simulink model "TemperatureControlledSystem"  (R2023b)
settings: Solver=FixedStepAuto  StartTime=0.0  StopTime=100  FixedStep=0.001  RelTol=1e-3
values from neighbouring files (symbols this model uses):
  TEMPMAX = 25.0    [temperatureControlledSystem.sldd]
  TEMPMIN = 10.0    [temperatureControlledSystem.sldd]
  TIMER = 5.0    [temperatureControlledSystem.sldd]
settings Model: DataDictionary=temperatureControlledSystem.sldd  Creator=dhabe  LastModifiedBy=dhabe
settings OptimizationCC: DefaultParameterBehavior=Inlined  EnhancedBackFolding=on  PassReuseOutputArgsAs=Individual arguments  ZeroExternalMemoryAtStartup=off  ZeroInternalMemoryAtStartup=off  OptimizeBlockOrder=speed  DifferentSizesBufferReuse=on  OptimizationCustomize=off  EfficientTunableParamExpr=on
settings DebuggingCC: ParameterTunabilityLossMsg=error
settings HardwareCC: ProdBitPerPointer=32  ProdBitPerSizeT=32  ProdBitPerPtrDiffT=32  ProdLargestAtomicFloat=None  ProdWordSize=32  ProdHWDeviceType=Atmel->AVR (32-bit)
settings SFSimCC: MATLABDynamicMemAlloc=off
settings RTWCC: Description=Embedded Coder  SystemTargetFile=ert.tlc  PackageGeneratedCodeAndArtifacts=on  TemplateMakefile=ert_default_tmf  PortableWordSizes=on
settings CodeAppCC: ForceParamTrailComments=on  IgnoreCustomStorageClasses=off  OperatorAnnotations=on  SimulinkDataObjDesc=on  SFDataObjDesc=on  InsertBlockDesc=on
settings ERTTargetCC: TargetLangStandard=C99 (ISO)  GenerateSampleERTMain=on  InlinedParameterPlacement=NonHierarchical  ERTCustomFileTemplate=example_file_process.tlc
settings ConfigComp: CovMetricSettings=dcmwe

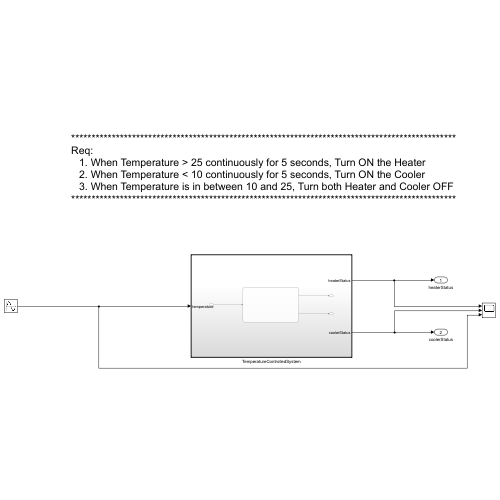
[thumbnail: Simulink's stored preview of the top-level diagram]
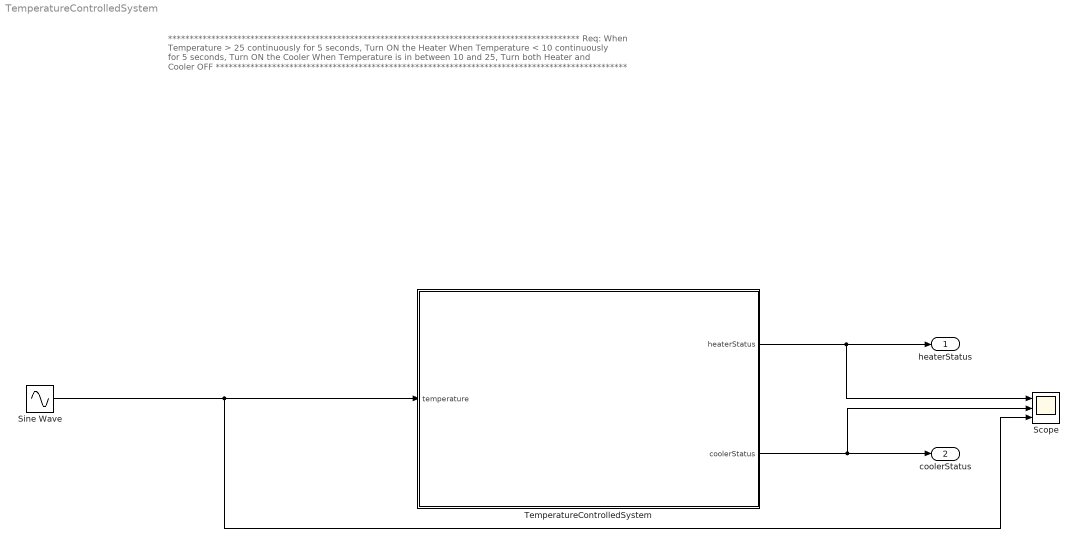
== system TemperatureControlledSystem ==
  note: ***********************************************************************************************
      | Req:
      | When Temperature > 25 continuously for 5 seconds, Turn ON the Heater
      | When Temperature < 10 continuously for 5 seconds, Turn ON the Cooler
      | When Temperature is in between 10 and 25, Turn both Heater and Cooler OFF
      | ***********************************************************************************************
  Scope : Scope  NumInputPorts=3
  Sine Wave : Sin  Amplitude=30  Frequency=0.1  SampleTime=0
  TemperatureControlledSystem : Subsystem  TreatAsAtomicUnit=on
  heaterStatus : Outport
  coolerStatus : Outport  Port=2
  wires:
  TemperatureControlledSystem/1(heaterStatus) -> Scope/1, heaterStatus/1
  TemperatureControlledSystem/2(coolerStatus) -> Scope/2, coolerStatus/1
  Sine Wave/1 -> Scope/3, TemperatureControlledSystem/1(temperature)

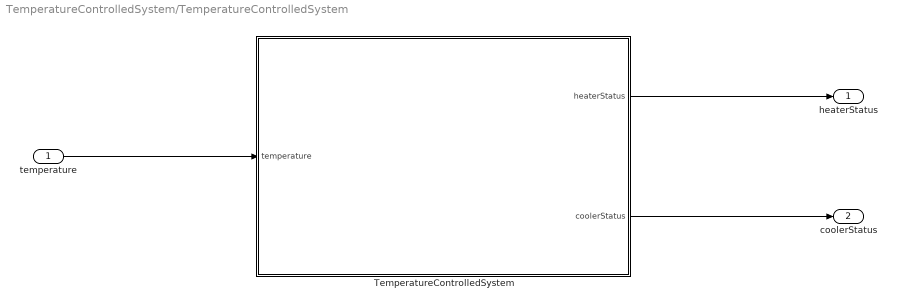
== system TemperatureControlledSystem/TemperatureControlledSystem ==
  temperature : Inport
  TemperatureControlledSystem : Stateflow chart  TreatAsAtomicUnit=on
  heaterStatus : Outport
  coolerStatus : Outport  Port=2
  wires:
  TemperatureControlledSystem/2(coolerStatus) -> coolerStatus/1
  temperature/1 -> TemperatureControlledSystem/1(temperature)
  TemperatureControlledSystem/1(heaterStatus) -> heaterStatus/1

== stateflow chart TemperatureControlledSystem/TemperatureControlledSystem ==
  settings: executeAtInitialization=1
  note: OFF = 0, ON = 1, TEMPMIN = 10, TEMPMAX = 25, TIMER = 5
  state IDLE
    en: heaterStatus = OFF, coolerStatus = OFF;
  state HEATERCONTROL
    en: heaterStatus = ON;
  state COOLERCONTROL
    en: coolerStatus = ON;
  (default) -> IDLE
  HEATERCONTROL -> IDLE : [temperature >= TEMPMIN]
  IDLE -> HEATERCONTROL [order 1] : [duration(temperature < TEMPMIN, sec) >= TIMER]
  COOLERCONTROL -> IDLE : [temperature <= TEMPMAX]
  IDLE -> COOLERCONTROL [order 2] : [duration(temperature > TEMPMAX, sec) >= TIMER]
  data: temperature input; heaterStatus output =0; coolerStatus output =0; OFF parameter; ON parameter; TEMPMAX parameter; TEMPMIN parameter; TIMER parameter
